simulink model "Lateral"  (R2025b)
settings: Solver=ode45  StartTime=0.0  StopTime=2.5  MinStep=0.00001  RelTol=1e-3
undefined symbols (not defined in the file): car, rad, s, Tau_1, Tau_2, Tau_3, Tau_4
libraries: aerolibconvert2 x3, simulink_extras x1, simulink x1
(part 3 of 3)

== matlab function Lateral/Longitudinal dynamics/Jr/MATLAB Function ==
  data: gear input; Jr_tot output; car input
function Jr_tot  = Jr(gear, car)

if gear == 1 
    Jr_tot = car.Jr_tot_1;
elseif gear == 2 
    Jr_tot = car.Jr_tot_2;
elseif gear == 3 
    Jr_tot = car.Jr_tot_3;
elseif gear == 4
    Jr_tot = car.Jr_tot_4;
else  
    Jr_tot = car.Jr_tot_0;
end

== matlab function Lateral/Longitudinal dynamics/delta_ Fx solver/RR ==
  data: Fx_ICE input; Fx_tyre input; delta_Fx_RR output
function delta_Fx_RR  = fcn(Fx_ICE, Fx_tyre)

delta_Fx_RR = Fx_ICE - Fx_tyre;

== matlab function Lateral/Longitudinal dynamics/Kinematics/Subsystem/MATLAB Function ==
  data: x input; dx output; M_pitch input; car input; c_FR input; c_RR input; c_FL input; c_RL input
function dx = Model7DOF(x, M_pitch, car, c_FR, c_RR, c_FL, c_RL)

q  = x(1:7);      % [heave; pitch; roll; z_ufl; z_ufr; z_url; z_urr]
dq = x(8:14);

ms  = car.m_sprung;
Iyy = car.Iyy;
Ixx = car.Ixx;
muf = car.m_unsprung_F;
mur = car.m_unsprung_R;

lf   = car.lf;    % distanza CG → asse anteriore
lr   = car.lr;    % distanza CG → asse posteriore
tf  = car.tf;   % carreggiata anteriore
tr  = car.tr;   % carreggiata posteriore

%sistemare se si vuole mettere differenziato sui 4 corners
ksf = car.k_spring_front * 1000 * car.IR_spring_front^2 + car.k_flexure * 1000; %sistemare con IR che cambia
ksr = car.k_spring_rear * 1000 * car.IR_spring_rear^2; %sistemare con IR che cambia
ktf = car.k_tyre * 1000;
ktr = car.k_tyre * 1000;

csf = c_FR * car.IR_spring_front^2; %sistemare
csr = c_RR * car.IR_spring_rear^2; %sistemare

M = diag([ms, Iyy, Ixx, muf, muf, mur, mur]);

K = [ 2*(ksf + ksr)      2*(lr*ksr-lf*ksf)       0          -ksf       -ksf       -ksr       -ksr;
      2*(lr*ksr-lf*ksf)    2*(lf^2*ksf+lr^2*ksr)  0           lf*ksf     lf*ksf      -lr*ksr     -lr*ksr;
      0                 0                 2*(tf^2*ksf+tr^2*ksr) -tf*ksf   tf*ksf   -tr*ksr   tr*ksr;
     -ksf               lf*ksf            -tf*ksf       ksf+ktf       0           0         0;
     -ksf               lf*ksf             tf*ksf       0             ksf+ktf     0         0;
     -ksr              -lr*ksr            -tr*ksr       0             0           ksr+ktr   0;
     -ksr              -lr*ksr             tr*ksr       0             0           0         ksr+ktr ];


C = [ 2*(csf + csr)      2*(lr*csr-lf*csf)        0         -csf       -csf       -csr       -csr;
      2*(lr*csr-lf*csf)    2*(lf^2*csf+lr^2*csr)   0          lf*csf     lf*csf     -lr*csr     -lr*csr;
      0                  0                 2*(tf^2*csf+tr^2*csr) -tf*csf   tf*csf  -tr*csr    tr*csr;
     -csf               lf*csf           -tf*csf       csf      0       0         0;
     -csf               lf*csf            tf*csf       0        csf     0         0;
     -csr              -lr*csr           -tr*csr       0         0       csr       0;
     -csr              -lr*csr            tr*csr       0         0        0        csr ];


F = [0; M_pitch; 0; 0; 0; 0; 0];

ddq = M \ (F - C*dq - K*q);

dx = zeros(14,1);
dx(1:7)   = dq;
dx(8:14)  = ddq;

end

== matlab function Lateral/Longitudinal dynamics/Fx powertrain calculation/RR ==
  data: Fx_ICE_RR output; T input; T_b input; ax input; Fz input; J_r input; car input; delta_z_tyre_RR input
function Fx_ICE_RR = fcn( T, T_b,ax, Fz, J_r, car, delta_z_tyre_RR)

Fx_ICE_RR = ( T - T_b - Fz * car.delta - J_r * ax / ( car.R - delta_z_tyre_RR ) ) / ( car.R - delta_z_tyre_RR ) ; %N; % J - parameter for each tyre - J_f & J_r

== matlab function Lateral/Longitudinal dynamics/Fx powertrain calculation/FR ==
  data: Fx_EM_FR output; T input; T_b input; Fz input; ax input; car input; delta_z_tyre_FR input
function Fx_EM_FR = fcn( T, T_b,Fz, ax, car, delta_z_tyre_FR )

Fx_EM_FR = ( T - T_b - Fz * car.delta - car.J_f * ax / ( car.R - delta_z_tyre_FR ) ) / ( car.R - delta_z_tyre_FR ) ; %N % J - parameter for each tyre - J_f & J_r

== matlab function Lateral/Longitudinal dynamics/Fx powertrain calculation/RL ==
  data: T input; T_b input; Fz input; ax input; J_r input; car input; Fx_ICE_RL output; delta_z_tyre_RL input
function Fx_ICE_RL = fcn( T, T_b, Fz, ax, J_r, car, delta_z_tyre_RL)

Fx_ICE_RL = ( T - T_b - Fz * car.delta - J_r * ax / ( car.R - delta_z_tyre_RL ) ) / ( car.R - delta_z_tyre_RL ) ; %N % J - parameter for each tyre - J_f & J_r

== matlab function Lateral/Longitudinal dynamics/delta_ Fx solver/RL ==
  data: Fx_ICE input; Fx_tyre input; delta_Fx_RL output
function delta_Fx_RL  = fcn(Fx_ICE, Fx_tyre)

delta_Fx_RL = Fx_ICE - Fx_tyre;

== matlab function Lateral/Longitudinal dynamics/delta_ Fx solver/FR ==
  data: Fx_EM input; Fx_tyre input; delta_Fx_FR output
function delta_Fx_FR  = fcn(Fx_EM, Fx_tyre)

delta_Fx_FR = Fx_EM - Fx_tyre ;

== matlab function Lateral/Longitudinal dynamics/delta_ Fx solver/FL ==
  data: Fx_EM input; Fx_tyre input; delta_Fx_FL output
function delta_Fx_FL  = fcn(Fx_EM, Fx_tyre)

delta_Fx_FL = Fx_EM - Fx_tyre;

== matlab function Lateral/Longitudinal dynamics/slip_tyres/FR ==
  data: delta_Fx_front input; delta_z_tyre_FR input; w_dot_slip_FR output; car input; R_def output
function [w_dot_slip_FR, R_def]  = slip(delta_Fx_front, delta_z_tyre_FR, car)

R_def = car.R - delta_z_tyre_FR;
w_dot_slip_FR = (delta_Fx_front * (R_def)) / car.J_f; %rad/s^2

== matlab function Lateral/Longitudinal dynamics/slip_tyres/FL ==
  data: delta_Fx_front input; delta_z_tyre_FL input; w_dot_slip_FL output; car input; R_def output
function [w_dot_slip_FL, R_def]  = slip(delta_Fx_front, delta_z_tyre_FL, car)

R_def = car.R - delta_z_tyre_FL;
w_dot_slip_FL = delta_Fx_front * (R_def) / car.J_f;

== matlab function Lateral/Tyres/Lateral forces/Front Right ==
  data: car input; SA input; Fy_FR output; Fz input; camber input
function Fy_FR = fcn(car,SA,Fz,camber)

%function Fy = fcn(SA,tyre,p,Fz,camber)
%if the tyre used is 'Hoosier_16x75x10_LCO_7_in_rim.tir' the sign of camber
%must be inverted because the .tir file is referring to a "right" tyre

%coefficienti dal file tir
Fz0 = car.tyre_Fz0;
%if Fz0 == 0, Fz0 = max(1, Fz); end
dfz = (Fz - Fz0)/Fz0;

pi0 = car.tyre_pi0;  % Pa nominale
dpi = (car.tyre_pressure_front - pi0)/pi0;
   
Cy1 = car.tyre_Cy1;
Dy1 = car.tyre_Dy1;
Dy2 = car.tyre_Dy2;
Dy3 = car.tyre_Dy3;
Ey1 = car.tyre_Ey1;
Ey2 = car.tyre_Ey2;
Ey3 = car.tyre_Ey3;
Ey4 = car.tyre_Ey4;
Ky1 = car.tyre_Ky1;
Ky2 = car.tyre_Ky2;
Ky3 = car.tyre_Ky3;
Hy1 = car.tyre_Hy1;
Hy2 = car.tyre_Hy2;
Hy3 = car.tyre_Hy3;
Vy1 = car.tyre_Vy1;
Vy2 = car.tyre_Vy2;
Vy3 = car.tyre_Vy3;
Vy4 = car.tyre_Vy4;
py1 = car.tyre_py1;
py2 = car.tyre_py2;
py3 = car.tyre_py3;
py4 = car.tyre_py4;
lmuy = car.tyre_lmuy;

%formule PAC2002 per il puro laterale
gamma = camber * pi/180;

% alpha = SA * pi/180;

alpha = SA;

mu = (Dy1 + Dy2 * dfz) * (1 - Dy3 * (gamma^2)) * (1 + py3 * dpi + py4 * dpi^2) * lmuy;

D = mu * Fz;

C = Cy1;

K0 = Ky1 * Fz0 * (1 + py1 * dpi) * sin(2 * atan(Fz / (Ky2 * Fz0 * (1 + py2 * dpi))));

K = K0 * (1 - Ky3 * abs(gamma));

B = K / (C * D + eps);

SH = Hy1 + Hy2 * dfz + Hy3 * gamma;

alpha  = alpha + SH;

E  = (Ey1 + Ey2 * dfz) * (1 - (Ey3 + Ey4 * gamma) * sign(alpha));

SV = Fz * ((Vy1 + Vy2 * dfz) + (Vy3 + Vy4 * dfz) * gamma);

Fy0 = D * sin(C * atan(B * alpha - E * (B * alpha - atan(B * alpha))));

Fy_FR = Fy0 + SV;

== matlab function Lateral/Longitudinal dynamics/slip_tyres/RL ==
  data: delta_Fx_rear input; w_dot_slip_RL output; delta_z_tyre_RL input; J_r input; car input; R_def output
function [w_dot_slip_RL, R_def]  = slip(delta_Fx_rear, delta_z_tyre_RL, J_r, car)

R_def = car.R - delta_z_tyre_RL;
w_dot_slip_RL = delta_Fx_rear * (R_def) / ( J_r );

== matlab function Lateral/Longitudinal dynamics/Kinematics/Subsystem/Damper FL/MATLAB Function ==
  data: x_dot input; x_dot_comp output; x_dot_reb output
function [ x_dot_comp , x_dot_reb ] = conv_x_dot(x_dot)

if x_dot > 0 
    x_dot_comp = x_dot; 
    x_dot_reb = 0;
else 
    x_dot_comp = 0;
    x_dot_reb = - x_dot;
end

== matlab function Lateral/Longitudinal dynamics/Kinematics/Subsystem/Damper RL/MATLAB Function ==
  data: x_dot input; x_dot_comp output; x_dot_reb output
function [ x_dot_comp , x_dot_reb ] = conv_x_dot(x_dot)

if x_dot > 0 
    x_dot_comp = x_dot; 
    x_dot_reb = 0;
else 
    x_dot_comp = 0;
    x_dot_reb = - x_dot;
end

== matlab function Lateral/Longitudinal dynamics/Kinematics/Subsystem/Damper FR/if stetement ==
  data: x_dot input; x_dot_comp output; x_dot_reb output
function [ x_dot_comp , x_dot_reb ] = conv_x_dot(x_dot)

if x_dot > 0 
    x_dot_comp = x_dot; 
    x_dot_reb = 0;
else 
    x_dot_comp = 0;
    x_dot_reb = - x_dot;
end

== matlab function Lateral/Longitudinal dynamics/Kinematics/Subsystem/Damper RR/MATLAB Function ==
  data: x_dot input; x_dot_comp output; x_dot_reb output
function [ x_dot_comp , x_dot_reb ] = conv_x_dot(x_dot)

if x_dot > 0 
    x_dot_comp = x_dot; 
    x_dot_reb = 0;
else 
    x_dot_comp = 0;
    x_dot_reb = - x_dot;
end

== matlab function Lateral/Longitudinal dynamics/Kinematics/Subsystem/damper velocity calculator ==
  data: car input; x input; x_dot_FR output; x_dot_FL output; x_dot_RL output; x_dot_RR output
function [x_dot_FR, x_dot_FL, x_dot_RL, x_dot_RR] = x_dot(car, x)

% Front speed: velocità unsprung - velocità sprung + (front wheelbase * velocità di pitch)

% Rear speed: velocità unsprung - velocità sprung - (rear wheelbase * velocità di pitch)

x_dot_FL = x(11) - x(8) + car.lf * x(9);
x_dot_FR = x(12) - x(8) + car.lf * x(9);

x_dot_RL = x(13) - x(8) + car.lr * x(9);
x_dot_RR = x(14) - x(8) - car.lr * x(9);

end

== matlab function Lateral/Longitudinal dynamics/slip_tyres/RR ==
  data: delta_Fx_rear input; w_dot_slip_RR output; delta_z_tyre_RR input; J_r input; car input; R_def output
function [w_dot_slip_RR, R_def]  = slip(delta_Fx_rear, delta_z_tyre_RR, J_r,car)

R_def = car.R - delta_z_tyre_RR;
w_dot_slip_RR = delta_Fx_rear * (R_def) / (J_r);

== matlab function Lateral/Solver/MATLAB Function ==
  data: delta input; a output; beta_dot output size=1; Fx input; Fy input; drag input; car input; beta input; yaw input; v input; yaw_dot output size=1
function [a, beta_dot, yaw_dot]  = fcn(delta, Fx, Fy, drag, car, beta, yaw, v)

a = 1/car.m * ((Fx(4) + Fx(3)) * cos(beta) + ((Fx(2) + Fx(1)) * cos(delta - beta)) + ((Fy(4) + Fy(3)) * sin(beta)) - ((Fy(1) + Fy(2)) * sin(delta - beta)) - drag);

yaw_dot = 1 / car.Izz * ((Fx(3) - Fx(4)) * car.tr / 2 - (Fy(3) + Fy(4))* car.lr + ((Fx(1) - Fx(2)) * cos(delta) + (Fy(2) - Fy(1)) * sin(delta)) * car.tf / 2 + ((Fy(2) + Fy(1)) * cos(delta) + (Fx(2) + Fx(1)) * sin(delta)) * car.lf);

if v < 0.05
    beta_dot = - yaw + 1 / (car.m * v + 0.1) * (-(Fx(3) + Fx(4)) * sin(beta) + (Fx(1) + Fx(2)) * sin(delta - beta) + (Fy(3) + Fy(4)) * cos(beta) + (Fy(1) + Fy(2)) * cos(delta - beta) + drag * tan(beta));
else
    beta_dot = - yaw + 1 / (car.m * v) * (-(Fx(3) + Fx(4)) * sin(beta) + (Fx(1) + Fx(2)) * sin(delta - beta) + (Fy(3) + Fy(4)) * cos(beta) + (Fy(1) + Fy(2)) * cos(delta - beta) + drag * tan(beta));
end

== matlab function Lateral/Longitudinal dynamics/MATLAB Function ==
  data: delta input; SA_FR output; yaw input; car input; beta input; v input; SA_FL output; SA_RR output; SA_RL output
function [SA_FR, SA_FL, SA_RR, SA_RL] = fcn(delta, yaw, car, beta, v)


SA_FR =  delta - atan((car.lf * yaw + v * sin(beta)) / (v * cos(beta) + 0.5 * car.tf * yaw));
SA_FL =  delta - atan((car.lf * yaw + v * sin(beta)) / (v * cos(beta) - 0.5 * car.tf * yaw));
SA_RR =  atan((car.lr * yaw - v * sin(beta)) / (v * cos(beta) + 0.5 * car.tr * yaw));
SA_RL =  atan((car.lr * yaw - v * sin(beta)) / (v * cos(beta) - 0.5 * car.tr * yaw));

if isnan(SA_RL)
        SA_RL = 0;
end

if isnan(SA_RR)
        SA_RR = 0;
end

if isnan(SA_FR)
        SA_FR = 0;
end

if isnan(SA_FL)
        SA_FL = 0;
end

== matlab function Lateral/Powertrain/Driver model - gear selection1/MATLAB Function3 ==
  settings: updateMethod=DISCRETE
  data: gear_trigger output; car input; gear_out output; v input
function [gear_trigger, gear_out] = change_gear(car, v)

    persistent gear
    if isempty(gear)
        gear = 2;      % start in 2nd
    end

    R = car.R; %

    % thresholds
    v_thresh_up   = [0, 24.9444, 45];   % 1-2, 2-3, 3-4
    % v_thresh_down = [0, 15, 15];          % 2-1, 3-2, 4-3, i numeri sono a caso quindi da cambiare

    tau      = [13.8304, 9.9320, 8.5118, 7.4490];
    nGearMax = numel(tau);

    gear_trigger = 0;
    old_gear     = gear;   % save old gear
    gear_out     = old_gear;

    % - UPSHIFT
    if old_gear < nGearMax && v >= v_thresh_up(old_gear)
        gear = old_gear + 1;
        gear_trigger = 1;

    % % - DOWNSHIFT
    % elseif old_gear > 2 && v <= v_thresh_down(old_gear)
    %     gear = old_gear - 1;
    %     gear_trigger = -1;
    % end

    gear_out = gear;
end

== matlab function Lateral/Tyres/Lateral forces/Front Left ==
  data: car input; SA input; Fy_FL output; Fz input; camber input
function Fy_FL = fcn(car,SA,Fz,camber)

%function Fy = fcn(SA,tyre,p,Fz,camber)
%if the tyre used is 'Hoosier_16x75x10_LCO_7_in_rim.tir' the sign of camber
%must be inverted because the .tir file is referring to a "right" tyre

%coefficienti dal file tir

Fz0 = car.tyre_Fz0;
%if Fz0 == 0, Fz0 = max(1, Fz); end
dfz = (Fz - Fz0)/Fz0;

pi0 = car.tyre_pi0;  % Pa nominale
dpi = (car.tyre_pressure_front - pi0)/pi0;

Cy1 = car.tyre_Cy1;
Dy1 = car.tyre_Dy1;
Dy2 = car.tyre_Dy2;
Dy3 = car.tyre_Dy3;
Ey1 = car.tyre_Ey1;
Ey2 = car.tyre_Ey2;
Ey3 = car.tyre_Ey3;
Ey4 = car.tyre_Ey4;
Ky1 = car.tyre_Ky1;
Ky2 = car.tyre_Ky2;
Ky3 = car.tyre_Ky3;
Hy1 = car.tyre_Hy1;
Hy2 = car.tyre_Hy2;
Hy3 = car.tyre_Hy3;
Vy1 = car.tyre_Vy1;
Vy2 = car.tyre_Vy2;
Vy3 = car.tyre_Vy3;
Vy4 = car.tyre_Vy4;
py1 = car.tyre_py1;
py2 = car.tyre_py2;
py3 = car.tyre_py3;
py4 = car.tyre_py4;
lmuy = car.tyre_lmuy;


%formule PAC2002 per il puro laterale
gamma = camber * pi/180;

% alpha = SA * pi/180;

alpha = SA;

mu = (Dy1 + Dy2 * dfz) * (1 - Dy3 * (gamma^2)) * (1 + py3 * dpi + py4 * dpi^2) * lmuy;

D = mu * Fz;

C = Cy1;

K0 = Ky1 * Fz0 * (1 + py1 * dpi) * sin(2 * atan(Fz / (Ky2 * Fz0 * (1 + py2 * dpi))));

K = K0 * (1 - Ky3 * abs(gamma));

B = K / (C * D + eps);

SH = Hy1 + Hy2 * dfz + Hy3 * gamma;

alpha  = alpha + SH;

E  = (Ey1 + Ey2 * dfz) * (1 - (Ey3 + Ey4 * gamma) * sign(alpha));

SV = Fz * ((Vy1 + Vy2 * dfz) + (Vy3 + Vy4 * dfz) * gamma);

Fy0 = D * sin(C * atan(B * alpha - E * (B * alpha - atan(B * alpha))));

Fy_FL = Fy0 + SV;

== matlab function Lateral/Powertrain/MATLAB Function1 ==
  settings: updateMethod=DISCRETE
  data: T_RL_in input; T_RR_in input; T_RL_out output; trigger input; T_RR_out output; time input
function [T_RL_out,T_RR_out] = fcn(T_RL_in, T_RR_in, trigger, time)

persistent t_start is_active prev_trigger
if isempty(t_start)
    t_start     = 0;
    is_active   = false;
    prev_trigger = 0;
end

% Rileva fronte di salita del trigger
if trigger == 1 && prev_trigger == 0
    t_start   = time;     % istante in cui parte il taglio coppia
    is_active = true;
end

% Disattiva dopo 0.15 s
if is_active && (time - t_start >= 0.15)
    is_active = false;
end

% Aggiorna trigger precedente
prev_trigger = trigger;

% Logica di uscita
if is_active
    T_RL_out = 0;
    T_RR_out = 0;
else
    T_RL_out = T_RL_in;
    T_RR_out = T_RR_in;
end
end

== matlab function Lateral/Powertrain/MATLAB Function2 ==
  data: w_ICE input; T_clutch input; T_powertrain output; T_ICE input; w_rear input; abs_w output
function [T_powertrain, abs_w] = Clutch(w_ICE, T_clutch, T_ICE, w_rear)

abs_w = w_ICE - w_rear;

if abs_w < 50
    T_powertrain = T_ICE;
else 
    T_powertrain = T_clutch;
end

== matlab function Lateral/Powertrain/MATLAB Function4 ==
  data: abs_w input; next_lockout_state output; prev_lockout_state input
function next_lockout_state = clutch_lockout_logic(abs_w, prev_lockout_state)
%
% This function calculates the next state for the clutch lockout.
% Once abs_w drops below 50, the output becomes 0 and stays 0 forever.
%
% Inputs:
% abs_w: The current absolute wheel speed signal.
% prev_lockout_state: The previous output state (memory from Unit Delay).
%
% Output:
% next_lockout_state: The output value (0 when locked, otherwise abs_w).

% Check if we're already locked out from previous step
% If prev_lockout_state == 0, we're already locked (output stuck at 0)
already_locked = (prev_lockout_state == 0);

% Check current lockout condition
lockout_triggered = (abs_w < 50);

% ----------------- LATCHING LOGIC -----------------
% Output becomes 0 and stays 0 if:
% 1. We're already locked out (previous output was 0)
% OR
% 2. Lockout condition is triggered now (abs_w < 50)
if already_locked || lockout_triggered
    next_lockout_state = 0; % Output locked to 0 forever
else
    next_lockout_state = abs_w; % Normal operation
end

== matlab function Lateral/Tyres/Lateral forces/Rear Right ==
  data: car input; SA input; Fy_RR output; Fz input; camber input
function Fy_RR = fcn(car,SA,Fz,camber)

%function Fy = fcn(SA,tyre,p,Fz,camber)
%if the tyre used is 'Hoosier_16x75x10_LCO_7_in_rim.tir' the sign of camber
%must be inverted because the .tir file is referring to a "right" tyre

%coefficienti dal file tir
Fz0 = car.tyre_Fz0;
%if Fz0 == 0, Fz0 = max(1, Fz); end
dfz = (Fz - Fz0)/Fz0;

pi0 = car.tyre_pi0;  % Pa nominale
dpi = (car.tyre_pressure_rear - pi0)/pi0;

Cy1 = car.tyre_Cy1;
Dy1 = car.tyre_Dy1;
Dy2 = car.tyre_Dy2;
Dy3 = car.tyre_Dy3;
Ey1 = car.tyre_Ey1;
Ey2 = car.tyre_Ey2;
Ey3 = car.tyre_Ey3;
Ey4 = car.tyre_Ey4;
Ky1 = car.tyre_Ky1;
Ky2 = car.tyre_Ky2;
Ky3 = car.tyre_Ky3;
Hy1 = car.tyre_Hy1;
Hy2 = car.tyre_Hy2;
Hy3 = car.tyre_Hy3;
Vy1 = car.tyre_Vy1;
Vy2 = car.tyre_Vy2;
Vy3 = car.tyre_Vy3;
Vy4 = car.tyre_Vy4;
py1 = car.tyre_py1;
py2 = car.tyre_py2;
py3 = car.tyre_py3;
py4 = car.tyre_py4;
lmuy = car.tyre_lmuy;


%formule PAC2002 per il puro laterale
gamma = camber * pi/180;

% alpha = SA * pi/180;

alpha = SA;

mu = (Dy1 + Dy2 * dfz) * (1 - Dy3 * (gamma^2)) * (1 + py3 * dpi + py4 * dpi^2) * lmuy;

D = mu * Fz;

C = Cy1;

K0 = Ky1 * Fz0 * (1 + py1 * dpi) * sin(2 * atan(Fz / (Ky2 * Fz0 * (1 + py2 * dpi))));

K = K0 * (1 - Ky3 * abs(gamma));

B = K / (C * D + eps);

SH = Hy1 + Hy2 * dfz + Hy3 * gamma;

alpha  = alpha + SH;

E  = (Ey1 + Ey2 * dfz) * (1 - (Ey3 + Ey4 * gamma) * sign(alpha));

SV = Fz * ((Vy1 + Vy2 * dfz) + (Vy3 + Vy4 * dfz) * gamma);

Fy0 = D * sin(C * atan(B * alpha - E * (B * alpha - atan(B * alpha))));

Fy_RR = Fy0 + SV;

== matlab function Lateral/Tyres/Lateral forces/Rear Left ==
  data: car input; SA input; Fy_RL output; Fz input; camber input
function Fy_RL = fcn(car,SA,Fz,camber)

%function Fy = fcn(SA,tyre,p,Fz,camber)
%if the tyre used is 'Hoosier_16x75x10_LCO_7_in_rim.tir' the sign of camber
%must be inverted because the .tir file is referring to a "right" tyre

%coefficienti dal file tir
Fz0 = car.tyre_Fz0;
%if Fz0 == 0, Fz0 = max(1, Fz); end
dfz = (Fz - Fz0)/Fz0;

pi0 = car.tyre_pi0;  % Pa nominale
dpi = (car.tyre_pressure_rear - pi0)/pi0;

Cy1 = car.tyre_Cy1;
Dy1 = car.tyre_Dy1;
Dy2 = car.tyre_Dy2;
Dy3 = car.tyre_Dy3;
Ey1 = car.tyre_Ey1;
Ey2 = car.tyre_Ey2;
Ey3 = car.tyre_Ey3;
Ey4 = car.tyre_Ey4;
Ky1 = car.tyre_Ky1;
Ky2 = car.tyre_Ky2;
Ky3 = car.tyre_Ky3;
Hy1 = car.tyre_Hy1;
Hy2 = car.tyre_Hy2;
Hy3 = car.tyre_Hy3;
Vy1 = car.tyre_Vy1;
Vy2 = car.tyre_Vy2;
Vy3 = car.tyre_Vy3;
Vy4 = car.tyre_Vy4;
py1 = car.tyre_py1;
py2 = car.tyre_py2;
py3 = car.tyre_py3;
py4 = car.tyre_py4;
lmuy = car.tyre_lmuy;

%formule PAC2002 per il puro laterale
gamma = camber * pi/180;

% alpha = SA * pi/180;

alpha = SA;

mu = (Dy1 + Dy2 * dfz) * (1 - Dy3 * (gamma^2)) * (1 + py3 * dpi + py4 * dpi^2) * lmuy;

D = mu * Fz;

C = Cy1;

K0 = Ky1 * Fz0 * (1 + py1 * dpi) * sin(2 * atan(Fz / (Ky2 * Fz0 * (1 + py2 * dpi))));

K = K0 * (1 - Ky3 * abs(gamma));

B = K / (C * D + eps);

SH = Hy1 + Hy2 * dfz + Hy3 * gamma;

alpha  = alpha + SH;

E  = (Ey1 + Ey2 * dfz) * (1 - (Ey3 + Ey4 * gamma) * sign(alpha));

SV = Fz * ((Vy1 + Vy2 * dfz) + (Vy3 + Vy4 * dfz) * gamma);

Fy0 = D * sin(C * atan(B * alpha - E * (B * alpha - atan(B * alpha))));

Fy_RL = Fy0 + SV;

== matlab function Lateral/Tyres/Longitudinal forces/Front Left ==
  data: car input; Fx_FL output; SR input; Fz input; camber input
function Fx_FL = fcn(car,SR,Fz,camber)

% PAC2002 puro longitudinale (Fx vs k)

     Fz0 = car.tyre_Fz0;
     if Fz0 == 0, Fz0 = max(1, Fz); end
    dfz = (Fz - Fz0)/Fz0;

    pi0 = car.tyre_pi0;  % Pa nominale
    dpi = (car.tyre_pressure_front - pi0)/pi0;
    
Cx1 = car.tyre_Cx1;
Dx1 = car.tyre_Dx1;
Dx2 = car.tyre_Dx2;
Dx3 = car.tyre_Dx3;
Ex1 = car.tyre_Ex1;
Ex2 = car.tyre_Ex2;
Ex3 = car.tyre_Ex3;
Ex4 = car.tyre_Ex4;
Kx1 = car.tyre_Kx1;
Kx2 = car.tyre_Kx2;
Kx3 = car.tyre_Kx3;
Hx1 = car.tyre_Hx1;
Hx2 = car.tyre_Hx2;
Vx1 = car.tyre_Vx1;
Vx2 = car.tyre_Vx2;
px1 = car.tyre_px1;
px2 = car.tyre_px2;
px3 = car.tyre_px3;
px4 = car.tyre_px4;
% lmux = car.tyre_lmux;


    gamma = camber * pi / 180;
    mu = (Dx1 + Dx2*dfz) * (1 - Dx3*(gamma^2)) * (1 + px3*dpi + px4*dpi^2)*car.scale_factor;
    % mu = 1.4;

    D = mu * Fz;
    C = Cx1;
    K = Fz * (Kx1 + Kx2*dfz) * exp(Kx3*dfz) * (1 + px1*dpi + px2*dpi^2);
    B = K / (C*D + eps);

    SH = Hx1 + Hx2*dfz;
    SR  = SR + SH;

    E  = (Ex1 + Ex2*dfz + Ex3*dfz^2) * (1 - Ex4*sign(SR));
    SV = Fz * (Vx1 + Vx2*dfz);

    Fx0 = D * sin( C * atan( B*SR - E*(B*SR - atan(B*SR)) ) );
    Fx_FL = Fx0 + SV;

== matlab function Lateral/Longitudinal dynamics/Fx equilibrium ==
  data: Drag output; Fz_FL output; ax input; vx input; Cx input; Cz input; delta_wb_front input; delta_wb_rear input; Jr_tot input; car input; ay input; Fz_RR output; Fz_RL output; Fz_FR output; delta_Fz output; beta input; M_inerzia output
function [Drag, Fz_FL, Fz_RR, Fz_RL, Fz_FR, delta_Fz, M_inerzia] = fx_equilibrium(ax, vx, Cx, Cz, delta_wb_front, delta_wb_rear, Jr_tot, car, ay, beta)

wb = car.wb0 + delta_wb_front + delta_wb_rear; %m

Downforce = 0.5 * car.rho * Cz * car.frontal_area * vx ^ 2 * (1 + tan(beta)); % downforce N
Drag = 0.5 * car.rho * Cx * car.frontal_area * vx ^ 2; % drag N
M_aero = Drag * (car.h_cp - car.h_cog) - Downforce * (car.lf - car.x_cp); %Nm

delta_Fz = Drag * car.h_cog / wb + M_aero / wb; %N
delta_Fz = delta_Fz / 2;

M_inerzia = car.m * ax * car.h_cog;
%J_f è di una singola ruota
%J_r totale da ruota a motore ICE
Fz_front = - Drag * car.h_cog / wb + (car.m * car.g + Downforce) * (car.lr + delta_wb_rear - car.delta) / wb - M_aero / wb - car.J_f*2* ax / (car.R * wb); %N  (verificare J_f*4 oppure J_f*2!!!!!!!!!!!)

Fz_rear = Drag * car.h_cog / wb + (car.m * car.g + Downforce) * (car.lf + delta_wb_front + car.delta) / wb + M_aero / wb + Jr_tot * ax / (car.R * wb); %N

% delta_Fz_lateral = car.m * ay * car.h_cog / ((car.tf + car.tr) / 2);
% 
% delta_Fz_lateral_front = car.k_roll_front / (car.k_roll_front + car.k_roll_rear) * delta_Fz_lateral;
% delta_Fz_lateral_rear = delta_Fz_lateral - delta_Fz_lateral_front;
% 
% Fz_FR = delta_Fz_lateral_front + Fz_front;
% Fz_FL = - delta_Fz_lateral_front + Fz_front;
% Fz_RR = delta_Fz_lateral_rear + Fz_rear;
% Fz_RL = - delta_Fz_lateral_rear + Fz_rear;

if Fz_front <= 0
    Fz_rear = Fz_rear + Fz_front;
    Fz_front = 0;
elseif Fz_rear <0 
    Fz_front = Fz_front + Fz_rear;
    Fz_rear = 0;
end

Fz_FR = Fz_front / 2;
Fz_FL = Fz_front / 2;
Fz_RR = Fz_rear / 2;
Fz_RL = Fz_rear / 2;
